simulink model "SimpleECU"  (R2026b)
undefined symbols (not defined in the file): CtrlEcuNidle, CtrlEcuRevLim, CtrlEcuStopTime
settings Model: Creator=The MathWorks, Inc.  LastModifiedBy=The MathWorks, Inc.

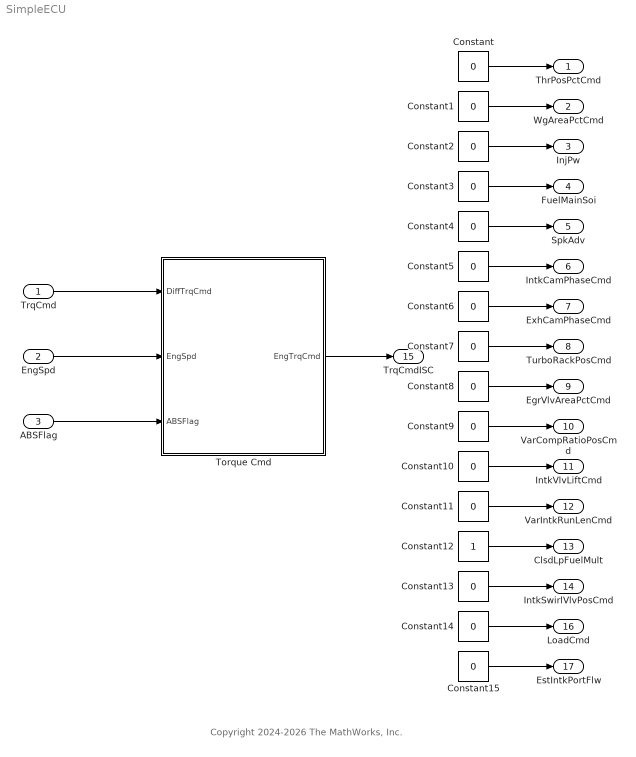
== system SimpleECU ==
  note: Copyright 2024-2026 The MathWorks, Inc.
  TrqCmd : Inport
  EngSpd : Inport  Port=2
  ABSFlag : Inport  Port=3  OutDataTypeStr=boolean
  Constant{,1..11,13..15} (15 alike) : Constant  Value=0  SampleTime=-1
  Constant12 : Constant  SampleTime=-1
  Torque Cmd : Subsystem
  ThrPosPctCmd : Outport  VectorParamsAs1DForOutWhenUnconnected=off
  WgAreaPctCmd : Outport  Port=2  VectorParamsAs1DForOutWhenUnconnected=off
  InjPw : Outport  Port=3  VectorParamsAs1DForOutWhenUnconnected=off
  FuelMainSoi : Outport  Port=4  Unit=deg  VectorParamsAs1DForOutWhenUnconnected=off
  SpkAdv : Outport  Port=5  VectorParamsAs1DForOutWhenUnconnected=off
  IntkCamPhaseCmd : Outport  Port=6  VectorParamsAs1DForOutWhenUnconnected=off
  ExhCamPhaseCmd : Outport  Port=7  VectorParamsAs1DForOutWhenUnconnected=off
  TurboRackPosCmd : Outport  Port=8  Unit=1  VectorParamsAs1DForOutWhenUnconnected=off
  EgrVlvAreaPctCmd : Outport  Port=9  Unit=%  VectorParamsAs1DForOutWhenUnconnected=off
  VarCompRatioPosCmd : Outport  Port=10  VectorParamsAs1DForOutWhenUnconnected=off
  IntkVlvLiftCmd : Outport  Port=11  VectorParamsAs1DForOutWhenUnconnected=off
  VarIntkRunLenCmd : Outport  Port=12  VectorParamsAs1DForOutWhenUnconnected=off
  ClsdLpFuelMult : Outport  Port=13  VectorParamsAs1DForOutWhenUnconnected=off
  IntkSwirlVlvPosCmd : Outport  Port=14  VectorParamsAs1DForOutWhenUnconnected=off
  TrqCmdISC : Outport  Port=15  VectorParamsAs1DForOutWhenUnconnected=off
  LoadCmd : Outport  Port=16  VectorParamsAs1DForOutWhenUnconnected=off
  EstIntkPortFlw : Outport  Port=17  VectorParamsAs1DForOutWhenUnconnected=off
  wires:
  ABSFlag/1 -> Torque Cmd/3(ABSFlag)
  Constant7/1 -> TurboRackPosCmd/1
  Constant4/1 -> SpkAdv/1
  Constant12/1 -> ClsdLpFuelMult/1
  Constant9/1 -> VarCompRatioPosCmd/1
  Constant14/1 -> LoadCmd/1
  Constant10/1 -> IntkVlvLiftCmd/1
  Constant13/1 -> IntkSwirlVlvPosCmd/1
  Torque Cmd/1(EngTrqCmd) -> TrqCmdISC/1
  Constant2/1 -> InjPw/1
  Constant15/1 -> EstIntkPortFlw/1
  Constant3/1 -> FuelMainSoi/1
  Constant/1 -> ThrPosPctCmd/1
  Constant5/1 -> IntkCamPhaseCmd/1
  Constant1/1 -> WgAreaPctCmd/1
  EngSpd/1 -> Torque Cmd/2(EngSpd)
  Constant11/1 -> VarIntkRunLenCmd/1
  Constant6/1 -> ExhCamPhaseCmd/1
  TrqCmd/1 -> Torque Cmd/1(DiffTrqCmd)
  Constant8/1 -> EgrVlvAreaPctCmd/1

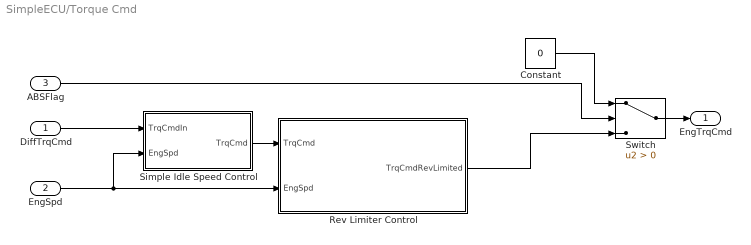
== system SimpleECU/Torque Cmd ==
  DiffTrqCmd : Inport
  EngSpd : Inport  Port=2  Unit=rpm
  ABSFlag : Inport  Port=3
  Constant : Constant  Value=0  SampleTime=-1
  Rev Limiter Control : Subsystem
  Simple Idle Speed Control : Subsystem
  Switch : Switch  Criteria=u2 > Threshold  ZeroCross=off  SaturateOnIntegerOverflow=off  InputSameDT=off
  EngTrqCmd : Outport
  wires:
  EngSpd/1 -> Simple Idle Speed Control/2(EngSpd), Rev Limiter Control/2(EngSpd)
  ABSFlag/1 -> Switch/2
  DiffTrqCmd/1 -> Simple Idle Speed Control/1(TrqCmdIn)
  Switch/1 -> EngTrqCmd/1
  Constant/1 -> Switch/1
  Rev Limiter Control/1(TrqCmdRevLimited) -> Switch/3
  Simple Idle Speed Control/1(TrqCmd) -> Rev Limiter Control/1(TrqCmd)

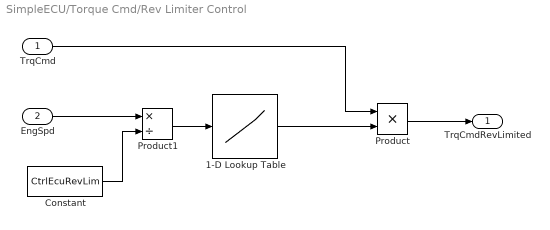
== system SimpleECU/Torque Cmd/Rev Limiter Control ==
  TrqCmd : Inport
  EngSpd : Inport  Port=2
  1-D Lookup Table : Lookup_n-D  NumberOfTableDimensions=1  BreakpointsForDimension1=[1 1.01]  Table=[1 0]  ExtrapMethod=Clip  InternalRulePriority=Speed  RndMeth=Simplest
  Constant : Constant  Value=CtrlEcuRevLim  SampleTime=-1
  Product : Product
  Product1 : Product  Inputs=*/
  TrqCmdRevLimited : Outport  VectorParamsAs1DForOutWhenUnconnected=off
  wires:
  EngSpd/1 -> Product1/1
  Product/1 -> TrqCmdRevLimited/1
  1-D Lookup Table/1 -> Product/2
  TrqCmd/1 -> Product/1
  Constant/1 -> Product1/2
  Product1/1 -> 1-D Lookup Table/1

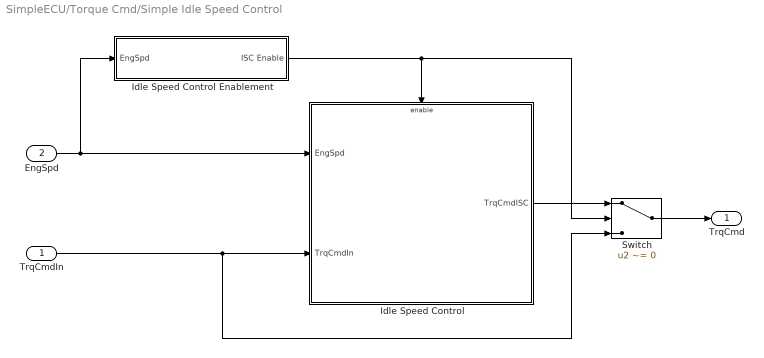
== system SimpleECU/Torque Cmd/Simple Idle Speed Control ==
  TrqCmdIn : Inport
  EngSpd : Inport  Port=2
  Idle Speed Control : Subsystem
  Idle Speed Control Enablement : Subsystem
  Switch : Switch  Criteria=u2 ~= 0  SaturateOnIntegerOverflow=off  InputSameDT=off
  TrqCmd : Outport  VectorParamsAs1DForOutWhenUnconnected=off
  wires:
  TrqCmdIn/1 -> Switch/3, Idle Speed Control/2(TrqCmdIn)
  EngSpd/1 -> Idle Speed Control Enablement/1(EngSpd), Idle Speed Control/1(EngSpd)
  Idle Speed Control Enablement/1(ISC Enable) -> Switch/2, Idle Speed Control/Enable
  Idle Speed Control/1(TrqCmdISC) -> Switch/1
  Switch/1 -> TrqCmd/1

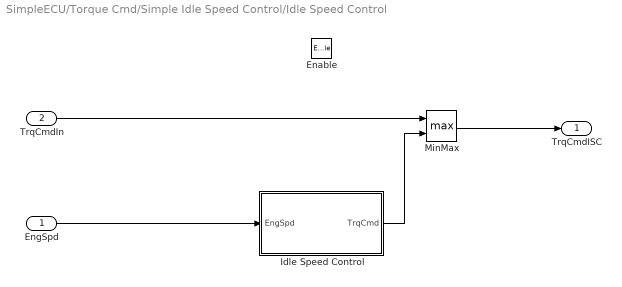
== system SimpleECU/Torque Cmd/Simple Idle Speed Control/Idle Speed Control ==
  EngSpd : Inport
  TrqCmdIn : Inport  Port=2
  Enable : EnablePort  StatesWhenEnabling=reset
  Idle Speed Control : Subsystem
  MinMax : MinMax  Function=max  Inputs=2
  TrqCmdISC : Outport
  wires:
  MinMax/1 -> TrqCmdISC/1
  TrqCmdIn/1 -> MinMax/1
  Idle Speed Control/1(TrqCmd) -> MinMax/2
  EngSpd/1 -> Idle Speed Control/1(EngSpd)

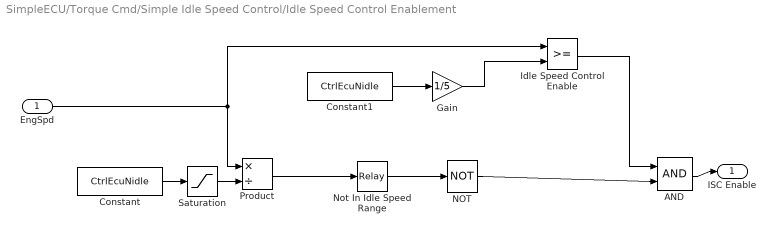
== system SimpleECU/Torque Cmd/Simple Idle Speed Control/Idle Speed Control Enablement ==
  EngSpd : Inport
  AND : Logic  IconShape=distinctive  AllPortsSameDT=off  OutDataTypeStr=boolean
  Constant : Constant  Value=CtrlEcuNidle
  Constant1 : Constant  Value=CtrlEcuNidle
  Gain : Gain  Gain=1/5
  Idle Speed Control Enable : RelationalOperator  OutDataTypeStr=boolean  RndMeth=Simplest  InputSameDT=off
  NOT : Logic  Operator=NOT  IconShape=distinctive  AllPortsSameDT=off  OutDataTypeStr=boolean
  Not In Idle Speed Range : Relay  OnSwitchValue=1.6  OffSwitchValue=1.3  OnOutputValue=true  OffOutputValue=false
  Product : Product  Inputs=*/
  Saturation : Saturate  UpperLimit=Inf  LowerLimit=1
  ISC Enable : Outport
  wires:
  Saturation/1 -> Product/2
  Constant/1 -> Saturation/1
  Product/1 -> Not In Idle Speed Range/1
  Not In Idle Speed Range/1 -> NOT/1
  NOT/1 -> AND/2
  Constant1/1 -> Gain/1
  Gain/1 -> Idle Speed Control Enable/2
  EngSpd/1 -> Idle Speed Control Enable/1, Product/1
  AND/1 -> ISC Enable/1
  Idle Speed Control Enable/1 -> AND/1

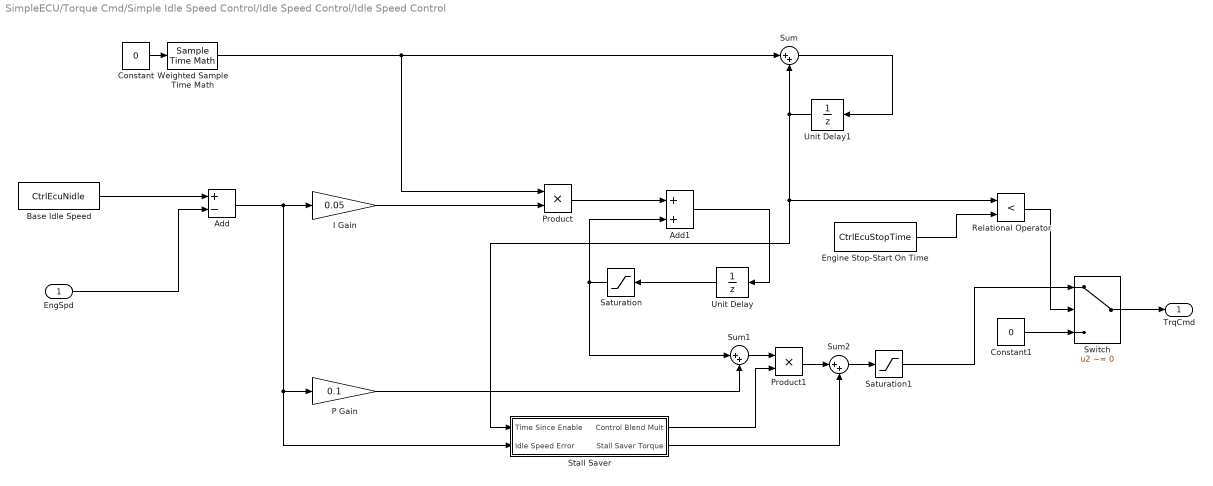
== system SimpleECU/Torque Cmd/Simple Idle Speed Control/Idle Speed Control/Idle Speed Control ==
  EngSpd : Inport
  Add : Sum  Inputs=+-
  Add1 : Sum
  Base Idle Speed : Constant  Value=CtrlEcuNidle
  Constant : Constant  Value=0
  Constant1 : Constant  Value=0
  Engine Stop-Start On Time : Constant  Value=CtrlEcuStopTime
  I Gain : Gain  Gain=0.05
  P Gain : Gain  Gain=0.1
  Product : Product
  Product1 : Product
  Relational Operator : RelationalOperator  Operator=<  OutDataTypeStr=boolean  RndMeth=Simplest  InputSameDT=off
  Saturation : Saturate  UpperLimit=50  LowerLimit=0
  Saturation1 : Saturate  UpperLimit=50  LowerLimit=0
  Stall Saver : Subsystem
  Sum : Sum  Inputs=|++
  Sum1 : Sum  Inputs=|++
  Sum2 : Sum  Inputs=|++
  Switch : Switch  Criteria=u2 ~= 0  SaturateOnIntegerOverflow=off  InputSameDT=off
  Unit Delay : UnitDelay  SampleTime=-1
  Unit Delay1 : UnitDelay  SampleTime=-1
  Weighted Sample Time Math : SampleTimeMath  TsampMathOp=Ts Only  weightValue=1
  TrqCmd : Outport  OutputWhenDisabled=reset  InitialOutput=1  VectorParamsAs1DForOutWhenUnconnected=off
  wires:
  Weighted Sample Time Math/1 -> Sum/1, Product/1
  Product/1 -> Add1/1
  Constant/1 -> Weighted Sample Time Math/1
  Saturation1/1 -> Switch/1
  Sum2/1 -> Saturation1/1
  P Gain/1 -> Sum1/2
  Saturation/1 -> Sum1/1, Add1/2
  I Gain/1 -> Product/2
  EngSpd/1 -> Add/2
  Add1/1 -> Unit Delay/1
  Base Idle Speed/1 -> Add/1
  Add/1 -> Stall Saver/2(Idle Speed Error), P Gain/1, I Gain/1
  Sum/1 -> Unit Delay1/1
  Unit Delay1/1 -> Stall Saver/1(Time Since Enable), Relational Operator/1, Sum/2
  Engine Stop-Start On Time/1 -> Relational Operator/2
  Relational Operator/1 -> Switch/2
  Switch/1 -> TrqCmd/1
  Constant1/1 -> Switch/3
  Stall Saver/2(Stall Saver Torque) -> Sum2/2
  Unit Delay/1 -> Saturation/1
  Sum1/1 -> Product1/1
  Stall Saver/1(Control Blend Mult) -> Product1/2
  Product1/1 -> Sum2/1

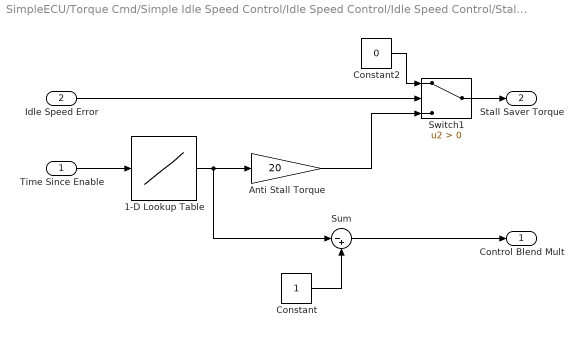
== system SimpleECU/Torque Cmd/Simple Idle Speed Control/Idle Speed Control/Idle Speed Control/Stall Saver ==
  Time Since Enable : Inport
  Idle Speed Error : Inport  Port=2
  1-D Lookup Table : Lookup_n-D  NumberOfTableDimensions=1  BreakpointsForDimension1=[0 0.75]  Table=[1 0]  ExtrapMethod=Clip  InternalRulePriority=Speed  RndMeth=Simplest
  Anti Stall Torque : Gain  Gain=20
  Constant : Constant
  Constant2 : Constant  Value=0
  Sum : Sum  Inputs=|-+
  Switch1 : Switch  Criteria=u2 > Threshold  SaturateOnIntegerOverflow=off  InputSameDT=off
  Control Blend Mult : Outport
  Stall Saver Torque : Outport  Port=2
  wires:
  Constant2/1 -> Switch1/1
  1-D Lookup Table/1 -> Sum/1, Anti Stall Torque/1
  Idle Speed Error/1 -> Switch1/2
  Switch1/1 -> Stall Saver Torque/1
  Time Since Enable/1 -> 1-D Lookup Table/1
  Anti Stall Torque/1 -> Switch1/3
  Constant/1 -> Sum/2
  Sum/1 -> Control Blend Mult/1
